simulink model "diagrama"  (R2015a)
settings: Solver=ode45  StartTime=0.0  StopTime=10.0  RelTol=1e-3
libraries: fuzblock x2
settings Model: Creator=IngAldair  LastModifiedBy=IngAldair

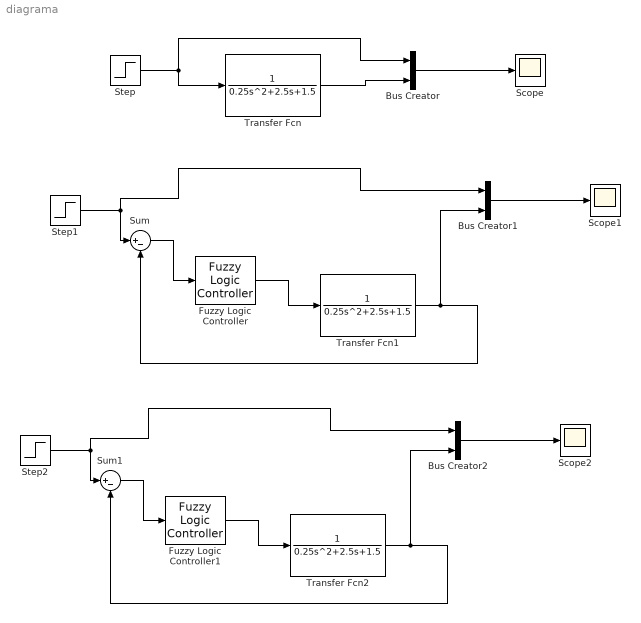
== system diagrama ==
  Bus Creator : BusCreator  Inputs=2
  Bus Creator1 : BusCreator  Inputs=2
  Bus Creator2 : BusCreator  Inputs=2
  Fuzzy Logic Controller : fuzblock/Fuzzy Logic  Controller  fis=controlador
  Fuzzy Logic Controller1 : fuzblock/Fuzzy Logic  Controller  fis=neurocontrolador
  Scope : Scope
  Scope1 : Scope
  Scope2 : Scope
      settings: SaveName=ScopeData2
  Step : Step  SampleTime=0
  Step1 : Step  SampleTime=0
  Step2 : Step  SampleTime=0
  Sum : Sum  Inputs=|+-
  Sum1 : Sum  Inputs=|+-
  Transfer Fcn : TransferFcn  Denominator=[0.25 2.5 1.5]
  Transfer Fcn1 : TransferFcn  Denominator=[0.25 2.5 1.5]
  Transfer Fcn2 : TransferFcn  Denominator=[0.25 2.5 1.5]
  wires:
  Step/1 -> Bus Creator/1, Transfer Fcn/1
  Transfer Fcn/1 -> Bus Creator/2
  Bus Creator/1 -> Scope/1
  Step1/1 -> Bus Creator1/1, Sum/1
  Bus Creator1/1 -> Scope1/1
  Fuzzy Logic Controller/1 -> Transfer Fcn1/1
  Sum/1 -> Fuzzy Logic Controller/1
  Transfer Fcn1/1 -> Bus Creator1/2, Sum/2
  Step2/1 -> Bus Creator2/1, Sum1/1
  Bus Creator2/1 -> Scope2/1
  Fuzzy Logic Controller1/1 -> Transfer Fcn2/1
  Sum1/1 -> Fuzzy Logic Controller1/1
  Transfer Fcn2/1 -> Bus Creator2/2, Sum1/2
